simulink model "step1"  (R2015a)
settings: Solver=ode45  StartTime=0.0  StopTime=1  RelTol=1e-3
values from neighbouring files (symbols this model uses):
  Dt = 1/(SampleRate*(N_in/N_out))    [DVBs2.m]    (also in DVBs2_2.m; Script.m)
  K_BCH = 51648    [DVBs2.m]    (also in DVBs2_2.m; Script.m)
  roll_off = 0.25    [DVBs2.m]    (also in DVBs2_2.m; Script.m)
undefined symbols (not defined in the file or in its folder): gcbh, rcfiltgaincompat
libraries: commblkcod2 x2, commrandsrc2 x1, commutil2 x1, commblkintrlv2 x1, commrflib2 x1, dspsigops x1, commdigbbndam3 x1, commfilt2 x1, commsequence2 x1
settings Model: Creator=Study  LastModifiedBy=Наталья
settings DataIOCC: SignalLoggingSaveFormat=ModelDataLogs
settings DebuggingCC: FcnCallInpInsideContextMsg=UseLocalSettings
settings GRTTargetCC: CombineOutputUpdateFcns=off  GRTInterface=on

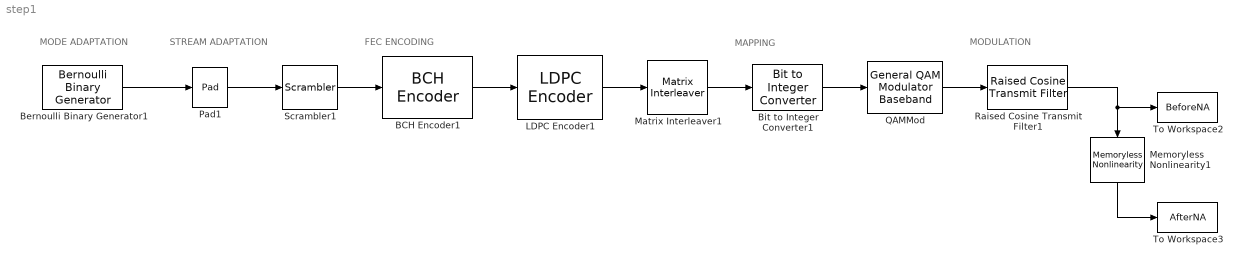
== system step1 ==
  note: MODULATION
  note: MAPPING
  note: FEC ENCODING
  note: STREAM ADAPTATION
  note: MODE ADAPTATION
  BCH Encoder1 : commblkcod2/BCH Encoder  n=N_BCH  k=K_BCH  specShortening=off  shortenedK=5  specGenPoly=on  genPoly=BCHGeneratorPoly  specPrimPoly=on  prPoly=BCHPrimitivePoly  specDisableGenCheck=off  specPuncture=off  punctVec=[ones(8,1); zeros(2,1)]
  Bernoulli Binary Generator1 : commrandsrc2/Bernoulli Binary Generator  P=0.5  seed=61  Ts=Dt  frameBased=on  sampPerFrame=N_in  orient=off  outDataType=double
  Bit to Integer Converter1 : commutil2/Bit to Integer Converter  nbits=NMOD  bitOrder=MSB first  signedOutputValues=Unsigned  outDtype=Inherit via internal rule  outDtypeSigned=Inherit via internal rule
  LDPC Encoder1 : commblkcod2/LDPC Encoder  ParityCheckMat=H
  Matrix Interleaver1 : commblkintrlv2/Matrix Interleaver  Nrows=Numofcols  Ncols=Numofrows
  Memoryless Nonlinearity1 : commrflib2/Memoryless Nonlinearity  model_select=Saleh model  linGaindB=0  GindB=0  iip3=30  am2pm=10  LPwrLimAMPM=10  UPwrLimAMPM=inf  amam=AM_AM  ampm=AM_PM  x=[8.1081 1.5413 6.5202 -0.0718]  y=[4.6645 2.0965 10.88 -0.003]  p=0.5  GoutdB=0  vsat=1
  Pad1 : dspsigops/Pad  padAlong=Columns  dimsToPad=1  valSrc=Specify via dialog  padVal=0  spec=Output size  padNumOutRowsSpecMethod=User-specified  numOutRows=K_BCH  padNumOutColsSpecMethod=User-specified  numOutCols=1  isVarDimsMode=off  padBeginning=0  padEnd=0  outSizeMode=User-specified  outSize=1  padSigAt=End  trunc_flag=None  roundingMode=Floor  overflowMode=off  truncOrWrapMode=Truncate  wrap_flag=None
  QAMMod : commdigbbndam3/General QAM Modulator Baseband  SigCon=[0.569019721201925+0.569019721201925i 0.777295394416168+0.208275673214243i 1.33112156537232+0.551368605544519i 1.4407956 -0.569019721201925+0.569019721201925i -0.777295394416168+0.208275673214243i -1.01879633906374+1.01879633906374i -1.33112156537232+0.551368605544519i 0.569019721201925-0.569019721201925i 0.777295394416168-0.208275673214244i 1.01879633906374-1.01879633906374i 1.33112156537232-0.55136860554452i -0.569019721201925-0.569019721201925i -0.777295394416168-0.208275673214243i -1.33112156537232-0.551368605544519i -1.4407956+1.76446571976559e-16i 0.208275673214243+0.777295394416168i 0.209198426912472+0.209198426912472i 0.551368605544519+1.33112156537232i 1.01879633906374+1.01879633906374i -0.208275673214243+0.777295394416168i -0.209198426912472+0.209198426912472i 8.82232859882795e-17+1.4407956i -0.551368605544519+1.33112156537232i 0.208275673214243-0.777295394416168i 0.209198426912472-0.209198426912472i -2.64669857964839e-16-1.4407956i 0.551368605544519-1.33112156537232i -0.208275673214244-0.777295394416168i -0.209198426912472-0.209198426912472i -0.55136860554452-1.33112156537232i -1.01879633906374-1.01879633906374i]  outDtype=double  outWordLen=16  outUDDataType=sfix(16)  outFracLenMode=Best precision  outFracLen=15
  Raised Cosine Transmit Filter1 : commfilt2/Raised Cosine Transmit Filter  filtType=Square root  filtSpan=2*(10)/2  currentFiltSpan=2*(10)/2  D=(2*(10)/2)/2  R=roll_off  sampMode=Mute  saveAsFlag=0  N=8  framing=Enforce single-rate processing  InputProcessing=Columns as channels (frame based)  checkGain=Normalized  filterGain=rcfiltgaincompat(gcbh)  checkCoeff=off  variableName=rcTxFilt1  launchFVT=off  roundingMode=Floor  overflowMode=off
  Scrambler1 : commsequence2/Scrambler  M=2  poly=[1 0 0 0 0 0 0 0 0 0 0 0 0 0 1 1]  iniStaSource=Dialog Parameter  ini_sta=[1 0 0 1 0 1 0 1 0 0 0 0 0 0 0]  resetViaPort=off
  To Workspace2 : ToWorkspace  VariableName=BeforeNA  SampleTime=-1
      settings: Save2DSignal=2-D array (concatenate along first dimension)
  To Workspace3 : ToWorkspace  VariableName=AfterNA  SampleTime=-1
      settings: Save2DSignal=2-D array (concatenate along first dimension)
  wires:
  Bernoulli Binary Generator1/1 -> Pad1/1
  Scrambler1/1 -> BCH Encoder1/1
  BCH Encoder1/1 -> LDPC Encoder1/1
  Pad1/1 -> Scrambler1/1
  Matrix Interleaver1/1 -> Bit to Integer Converter1/1
  Bit to Integer Converter1/1 -> QAMMod/1
  LDPC Encoder1/1 -> Matrix Interleaver1/1
  QAMMod/1 -> Raised Cosine Transmit Filter1/1
  Memoryless Nonlinearity1/1 -> To Workspace3/1
  Raised Cosine Transmit Filter1/1 -> To Workspace2/1, Memoryless Nonlinearity1/1
